simulink model "Use_Cases_N4_a"  (R2020b)
settings: Solver=ode3  StartTime=0.0  StopTime=inf  FixedStep=0.05  RelTol=1e-3
libraries: XBotBlockToolbox x3, simulink x1, Utilities x1

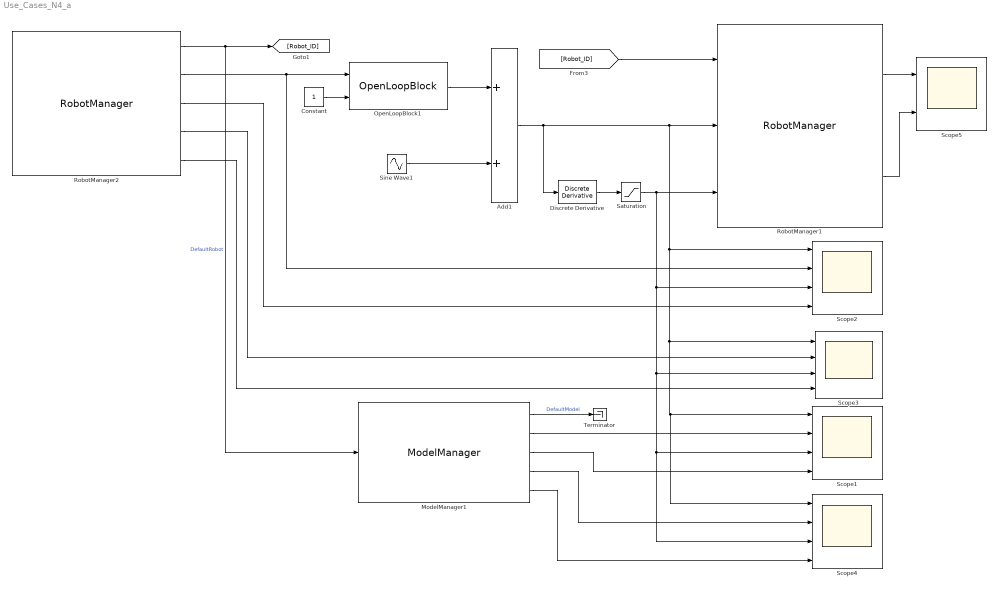
== system Use_Cases_N4_a ==
  Add1 : Sum
  Constant : Constant
  Discrete Derivative : simulink/Discrete/Discrete Derivative  gainval=1.0  ICPrevScaledInput=0.0  OutMin=[]  OutMax=[]  OutDataType=fixdt(1, 16)  OutScaling=2^-10  DoSatur=off
  ModelManager1 : XBotBlockToolbox/ModelManager  ModelName=DefaultModel  RobotName=DefaultRobot  UseExtModel=Off  SyncWithRobot=On  GetFloatingBaseList={}  SetFloatingBaseComponent=Off  GravityRequest=Off  ReadingsList={ 'qJ', 'qJdot', 'qJ_ref', 'qJdot_ref' }  MechanicalLimitsList={}  MechanicalLimitsCheck=Off  MechanicalLimitsEnforce=Off  SensorList={}  ReferencesList={}  OldModelName=DefaultModel
  OpenLoopBlock1 : Utilities/OpenLoopBlock  SystemSampleTime=-1  VariantActivationTime=update diagram  Latency=0  AutoFrameSizeCalculation=off
  RobotManager1 : XBotBlockToolbox/RobotManager  RobotName=DefaultRobot  ModelName=DefaultRobot  UseExtRobot=On  SyncWithModel=Off  ReadingsList={}  MechanicalLimitsList={}  MechanicalLimitsCheck=On  MechanicalLimitsEnforce=On  SensorList={}  ReferencesList={ 'qJ_ref', 'qJdot_ref' }  OldRobotName=DefaultRobot
  RobotManager2 : XBotBlockToolbox/RobotManager  RobotName=DefaultRobot  ModelName=DefaultModel  UseExtRobot=Off  SyncWithModel=Off  ReadingsList={ 'qJ', 'qJdot', 'qJ_ref', 'qJdot_ref' }  MechanicalLimitsList={}  MechanicalLimitsCheck=Off  MechanicalLimitsEnforce=Off  SensorList={}  ReferencesList={}  OldRobotName=DefaultRobot
  Saturation : Saturate  UpperLimit=0.2  LowerLimit=-0.2
  Scope{1..4} (4 alike) : Scope  NumInputPorts=4
  Scope5 : Scope  NumInputPorts=2
  Sine Wave1 : Sin  Amplitude=0.2  SampleTime=0
  Terminator : Terminator
  wires:
  RobotManager2/2 -> Scope2/2, OpenLoopBlock1/1
  Add1/1 -> RobotManager1/2, Scope3/1, Scope4/1, Scope1/1, Scope2/1, Discrete Derivative/1
  Discrete Derivative/1 -> Saturation/1
  [Robot_ID] -> RobotManager1/1
  Saturation/1 -> RobotManager1/3, Scope4/3, Scope1/3, Scope3/3, Scope2/3
  RobotManager2/3 -> Scope2/4
  Sine Wave1/1 -> Add1/2
  RobotManager2/5 -> Scope3/4
  RobotManager2/4 -> Scope3/2
  RobotManager2/1 -> ModelManager1/1, [Robot_ID]  "DefaultRobot"
  OpenLoopBlock1/1 -> Add1/1
  ModelManager1/1 -> Terminator/1  "DefaultModel"
  ModelManager1/2 -> Scope1/2
  ModelManager1/3 -> Scope1/4
  ModelManager1/4 -> Scope4/2
  ModelManager1/5 -> Scope4/4
  Constant/1 -> OpenLoopBlock1/2
  RobotManager1/1 -> Scope5/1
  RobotManager1/2 -> Scope5/2
